simulink subsystem "dynamics"  (R2023b)
settings: Solver=VariableStepAuto  StartTime=0.0  StopTime=10.0  RelTol=1e-3
undefined symbols (not defined in the file): a, b, Cf_rad, Cr_rad, Iz, raptor_xcp_function, totalMass, Vcg
libraries: Raptor_lib x39, dynamics_lib x11, cstblocks x1, mpclib x1
settings Model: Creator=serga  LastModifiedBy=serga
settings OptimizationCC: ReuseModelBlockBuffer=off

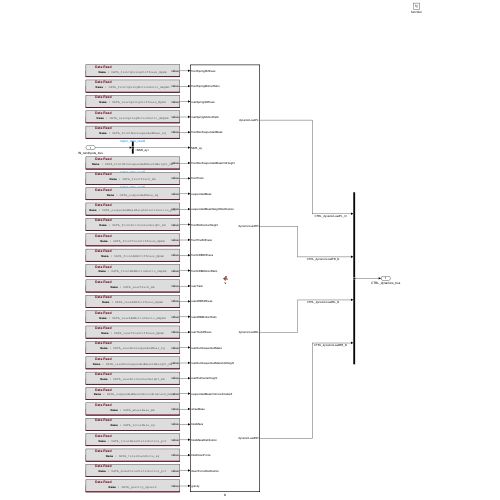
[thumbnail: Simulink's stored preview of the top-level diagram]
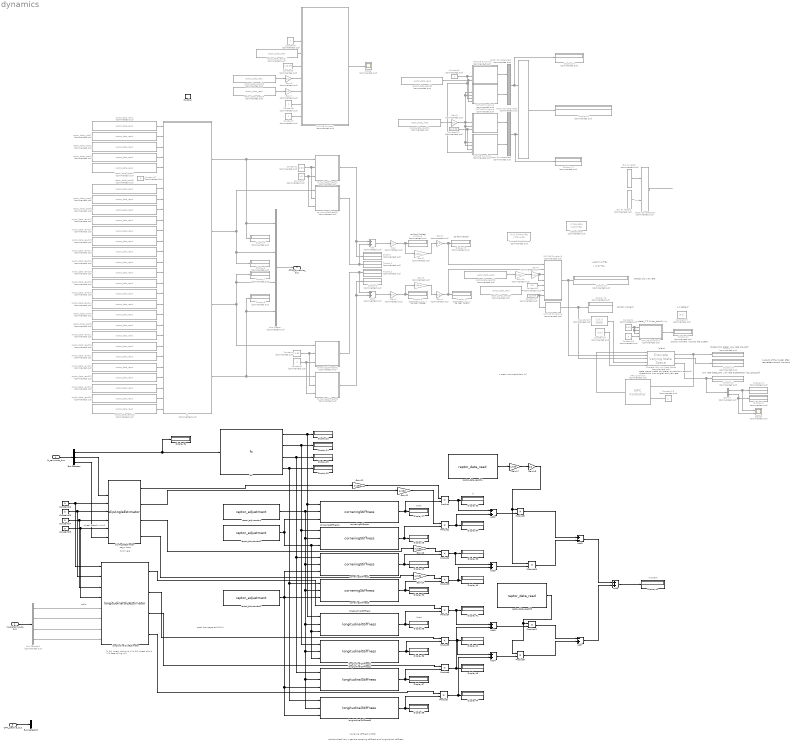
== system dynamics ==
  note: N
  note: moment
  note: peak tire usage at 0.3-0.4
  note: % full wheel lockup is -1
      | % full wheel slip is 1
      | % free rolling is 0
  note: rad/s
  note: wheel speed in km/h
  note: km/h here
  note: deg/s here
  note: double check how u get the cornering stiffness and longitudinal stiffness
  note: cornering stiffness = BCD
  note: outputs of the model after requested control moment
  note: "plant"
  note: state space model for lateral dynamics in terms of chassis slip (yaw angle) and yaw rate
  note: control moment, input to the system
  note: delta_T = Kr*psi_dot+Kv*vy
  note: chassis slip (beta), yaw rate (psi_dot)
  note: yaw rate (beta_dot), yaw rate acceleration (psi_dot_dot))
  note: u matrix as output from lu?
  note: y = Cx+Du
  note: x_dot = Ax+Bu
  note: control moment
  note: chassis slip
      | yaw rate
  note: ca rear (N/deg)
  note: ca front (N/deg)
  note: ca front (N/rad)
  note: ca rear (N/rad)
  note: u is delta_T
  note: N/rad
  note: N/rad
  IN_canInputs_bus : Inport
  IN_digitalInputs_bus : Inport  Port=2
  CTRL_tractive_bus : Inport  Port=3
  function : TriggerPort  TriggerType=function-call  VariantControl=(inherit)
  Add : Sum  Commented=on
  Add1 : Sum  Commented=on
  Add{2..5,8} (5 alike) : Sum
  Add6 : Sum  Inputs=+-
  Add7 : Sum  Inputs=-+
  Bus Creator : BusCreator  Commented=on  Inputs=4
  Bus Selector : BusSelector  OutputSignals=IN_can2Inputs_bus.CAN2_mm5_bus.CAN2_mm5_372_bus.MM5_ay,IN_can2Inputs_bus.CAN2_mm5_bus.CAN2_mm5_372_bus.MM5_yawRate,IN_can1Inputs_bus.CAN1_lws_bus.CAN1_lws_688_bus.LWS_angle
  Bus Selector1 : BusSelector  Commented=on  OutputSignals=IN_wheelSpeed_Bus.IN_wheelSpeedFL_bus.IN_wheelSpeedFL_radpsec,IN_wheelSpeed_Bus.IN_wheelSpeedFR_bus.IN_wheelSpeedFR_radpsec,IN_wheelSpeed_Bus.IN_wheelSpeedRL_bus.IN_wheelSpeedRL_radpsec,IN_wheelSpeed_Bus.IN_wheelSpeedRR_bus.IN_wheelSpeedRR_radpsec
  Bus Selector2 : BusSelector  OutputSignals=CTRL_vehicleSpeed_mph
  Bus to Vector : BusToVector  Commented=on
  Bus to Vector1 : BusToVector  Commented=on
  Constant : Constant  Commented=on  Value=0.83
  Constant{1,6..9,18} (6 alike) : Constant  Commented=on
  Constant10 : Constant  Commented=on  Value=113.95
  Constant11 : Constant  Commented=on  Value=113.95
  Constant12 : Constant  Commented=on  Value=15
  Constant13 : Constant  Commented=on  Value=[1 0; 0 10000]  VectorParams1D=off
  Constant14 : Constant  Commented=on  Value=[0;0]  VectorParams1D=off
  Constant15 : Constant  Commented=on  Value=[0.1]  VectorParams1D=off
  Constant16 : Constant  Commented=on  Value=3
  Constant17 : Constant  Commented=on  Value=0
  Constant2 : Constant  Commented=on  Value=0.83
  Constant{22..25} (4 alike) : Constant  Value=5
  Constant3 : Constant  Commented=on  Value=1.5
  Constant4 : Constant  Commented=on  Value=0.01
  Constant5 : Constant  Commented=on  Value=113.95
  Demux : Demux  Commented=on  Outputs=2
  Discrete State-Space : DiscreteStateSpace  Commented=on  SampleTime=-1
  Discrete Varying State Space : cstblocks/Linear Parameter Varying/Discrete Varying State Space  Commented=on  x0=0  Ts=-1  OutputX=on  OutputDX=on  Feedthrough=on
  Display{,1..22} (23 alike) : Display  Commented=on
  Display{23..31,33..45} (22 alike) : Display
  Gain : Gain  Commented=on  Gain=1/4
  Gain1 : Gain  Commented=on  Gain=1/4
  Gain10 : Gain  Commented=on  Gain=1/100
  Gain{11..14} (4 alike) : Gain  Gain=pi/180
  Gain17 : Gain  Gain=1/100
  Gain18 : Gain  Gain=1/2
  Gain2 : Gain  Commented=on  Gain=180/pi
  Gain3 : Gain  Commented=on  Gain=180/pi
  Gain{4..9} (6 alike) : Gain  Commented=on  Gain=1/2
  MATLAB Function : MATLAB Function  Commented=on  TreatAsAtomicUnit=on
  MATLAB Function1 : MATLAB Function  Commented=on  TreatAsAtomicUnit=on
  MATLAB Function2 : MATLAB Function  Commented=on  TreatAsAtomicUnit=on
  MATLAB Function3 : MATLAB Function  Commented=on  TreatAsAtomicUnit=on
  MATLAB Function4 : MATLAB Function  Commented=on  TreatAsAtomicUnit=on
  MATLAB Function5 : MATLAB Function  Commented=on  TreatAsAtomicUnit=on
  MATLAB Function6 : MATLAB Function  Commented=on  TreatAsAtomicUnit=on
  MATLAB Function7 : MATLAB Function  Commented=on  TreatAsAtomicUnit=on
  MPC Controller : mpclib/MPC Controller  Commented=on  SCDEnableBlockLinearizationSpecification=on  is_multiple=0  enable_value=0  return_u0=off  updateMPCinCallerWorkspace=on  md_inport=off  mv_inport=off  uref_inport=off  return_cost=off  return_mvseq=off  return_qpstatus=off  return_xseq=off  return_state=off  return_ovseq=off  state_inport=off  umin_inport=off  umax_inport=off  ymin_inport=off  ymax_inport=off  cc_inport=off  ywt_inport=off  uwt_inport=off  duwt_inport=off  rhoeps_inport=off  pm_inport=off  MaximumP=10  HorizonChoice=FixedHorizon  n_ts=0.1  n_p=10  n_mv=1  n_md=1  n_ud=0  n_mo=1  n_uo=0  BlockDataType=double  SampleTimeInherited=off  switch_inport=off
  Product{,1..11} (12 alike) : Product
  Scope : Scope  Commented=on
  Scope1 : Scope  Commented=on  NumInputPorts=2
  State-Space : StateSpace  Commented=on  A=[-(2*(Cf_rad+Cr_rad))/(Vcg*totalMass) -(2*(a*Cf_rad-b*Cr_rad))/(Vcg^2*totalMass)-1; -(2*(a*Cf_rad-2*b*Cr_rad))/Iz -(2*(a^2*Cf_rad-b^2*Cr_rad))/(Vcg*Iz)]  B=[0; 1/Iz]  C=[1 0; 0 1]  D=[0; 0]  InitialCondition=0
  Vector Concatenate : Concatenate  Commented=on  Mode=Multidimensional array  ConcatenateDimension=2
  Vector Concatenate2 : Concatenate  Commented=on
  Vector Concatenate3 : Concatenate  Commented=on
  Vector Concatenate4 : Concatenate  Commented=on  Mode=Multidimensional array  ConcatenateDimension=2
  corneringStiffness : dynamics_lib/corneringStiffness  pos='FL'
  corneringStiffness1 : dynamics_lib/corneringStiffness  pos='FR'
  corneringStiffness2 : dynamics_lib/corneringStiffness  pos='RL'
  corneringStiffness3 : dynamics_lib/corneringStiffness  pos='RR'
  corneringStiffnessFL : MATLAB Function  Commented=on  TreatAsAtomicUnit=on
  corneringStiffnessFR : MATLAB Function  Commented=on  TreatAsAtomicUnit=on
  corneringStiffnessRL : MATLAB Function  Commented=on  TreatAsAtomicUnit=on
  corneringStiffnessRR : MATLAB Function  Commented=on  TreatAsAtomicUnit=on
  fz : MATLAB Function  Commented=on  TreatAsAtomicUnit=on
  fz1 : dynamics_lib/fz  SystemSampleTime=-1  VariantActivationTime=update diagram  AllowFlexibleInterface=on  Latency=0  AutoFrameSizeCalculation=off
  longitudinalSlipEstimator : dynamics_lib/longitudinalSlipEstimator  SystemSampleTime=-1  VariantActivationTime=update diagram  AllowFlexibleInterface=on  Latency=0  AutoFrameSizeCalculation=off
  longitudinalStiffness : dynamics_lib/longitudinalStiffness  pos='FL'
  longitudinalStiffness1 : dynamics_lib/longitudinalStiffness  pos='FR'
  longitudinalStiffness2 : dynamics_lib/longitudinalStiffness  pos='RL'
  longitudinalStiffness3 : dynamics_lib/longitudinalStiffness  pos='RR'
  raptor_adjustment : Raptor_lib/Data Storage/raptor_adjustment  paramName='DATA_tirePressure_bar'  nameSource=Parameter  initValue=0.83  dataType=double  storage=Calibration  calDispType=Number  calEnum={'False', 'True'}  calGain=1.0  calOffset=0.0  calMax=inf  calMin=-inf  calFormat='-1'  calUnit=''  calHelp=''  calAccess=1  calFunction=raptor_xcp_function(gcb)  calDispHeaders=off  calColHeaders={'Col1' 'Col2' 'Col3'}  calRowHeaders={'Row1' 'Row2' 'Row3'}
      settings: SourceProductName=Raptor
  raptor_adjustment1 : Raptor_lib/Data Storage/raptor_adjustment  paramName='DATA_inclineAngleF_deg'  nameSource=Parameter  initValue=1.5  dataType=single  storage=Calibration  calDispType=Number  calEnum={'False', 'True'}  calGain=1.0  calOffset=0.0  calMax=inf  calMin=-inf  calFormat='-1'  calUnit=''  calHelp=''  calAccess=1  calFunction=raptor_xcp_function(gcb)  calDispHeaders=off  calColHeaders={'Col1' 'Col2' 'Col3'}  calRowHeaders={'Row1' 'Row2' 'Row3'}
      settings: SourceProductName=Raptor
  raptor_adjustment2 : Raptor_lib/Data Storage/raptor_adjustment  paramName='DATA_inclineAngleR_deg'  nameSource=Parameter  initValue=1  dataType=single  storage=Calibration  calDispType=Number  calEnum={'False', 'True'}  calGain=1.0  calOffset=0.0  calMax=inf  calMin=-inf  calFormat='-1'  calUnit=''  calHelp=''  calAccess=1  calFunction=raptor_xcp_function(gcb)  calDispHeaders=off  calColHeaders={'Col1' 'Col2' 'Col3'}  calRowHeaders={'Row1' 'Row2' 'Row3'}
      settings: SourceProductName=Raptor
  raptor_data_read : Raptor_lib/Data Storage/raptor_data_read  Commented=on  dataName='DATA_frontSpringStiffness_Npmm'  dataShape=Scalar  idxSource=Input  idxRow=1  idxCol=1
      settings: SourceProductName=Raptor
  raptor_data_read1 : Raptor_lib/Data Storage/raptor_data_read  Commented=on  dataName='DATA_rearSpringStiffness_Npmm'  dataShape=Scalar  idxSource=Input  idxRow=1  idxCol=1
      settings: SourceProductName=Raptor
  raptor_data_read10 : Raptor_lib/Data Storage/raptor_data_read  Commented=on  dataName='DATA_suspendedMassWeightDistribution_pct'  dataShape=Scalar  idxSource=Input  idxRow=1  idxCol=1
      settings: SourceProductName=Raptor
  raptor_data_read11 : Raptor_lib/Data Storage/raptor_data_read  Commented=on  dataName='DATA_frontRollCenterHeight_mm'  dataShape=Scalar  idxSource=Input  idxRow=1  idxCol=1
      settings: SourceProductName=Raptor
  raptor_data_read12 : Raptor_lib/Data Storage/raptor_data_read  Commented=on  dataName='DATA_rearRollCenterHeight_mm'  dataShape=Scalar  idxSource=Input  idxRow=1  idxCol=1
      settings: SourceProductName=Raptor
  raptor_data_read13 : Raptor_lib/Data Storage/raptor_data_read  Commented=on  dataName='DATA_frontTireStiffness_Npmm'  dataShape=Scalar  idxSource=Input  idxRow=1  idxCol=1
      settings: SourceProductName=Raptor
  raptor_data_read14 : Raptor_lib/Data Storage/raptor_data_read  Commented=on  dataName='DATA_rearTireStiffness_Npmm'  dataShape=Scalar  idxSource=Input  idxRow=1  idxCol=1
      settings: SourceProductName=Raptor
  raptor_data_read15 : Raptor_lib/Data Storage/raptor_data_read  Commented=on  dataName='DATA_rearARBStiffness_Npmm'  dataShape=Scalar  idxSource=Input  idxRow=1  idxCol=1
      settings: SourceProductName=Raptor
  raptor_data_read16 : Raptor_lib/Data Storage/raptor_data_read  Commented=on  dataName='DATA_frontARBMotionRatio_mmpmm'  dataShape=Scalar  idxSource=Input  idxRow=1  idxCol=1
      settings: SourceProductName=Raptor
  raptor_data_read17 : Raptor_lib/Data Storage/raptor_data_read  Commented=on  dataName='DATA_frontARBStiffness_Npmm'  dataShape=Scalar  idxSource=Input  idxRow=1  idxCol=1
      settings: SourceProductName=Raptor
  raptor_data_read18 : Raptor_lib/Data Storage/raptor_data_read  Commented=on  dataName='DATA_rearARBMotionRatio_mmpmm'  dataShape=Scalar  idxSource=Input  idxRow=1  idxCol=1
      settings: SourceProductName=Raptor
  raptor_data_read19 : Raptor_lib/Data Storage/raptor_data_read  Commented=on  dataName='DATA_rearTrack_mm'  dataShape=Scalar  idxSource=Input  idxRow=1  idxCol=1
      settings: SourceProductName=Raptor
  raptor_data_read2 : Raptor_lib/Data Storage/raptor_data_read  Commented=on  dataName='DATA_frontSpringMotionRatio_mmpmm'  dataShape=Scalar  idxSource=Input  idxRow=1  idxCol=1
      settings: SourceProductName=Raptor
  raptor_data_read20 : Raptor_lib/Data Storage/raptor_data_read  Commented=on  dataName='DATA_suspendedMassCGCoordinatesZ_mm'  dataShape=Scalar  idxSource=Input  idxRow=1  idxCol=1
      settings: SourceProductName=Raptor
  raptor_data_read{21,28..29,31..32} (5 alike) : Raptor_lib/Data Storage/raptor_data_read  Commented=on  dataName='DATA_wheelBase_mm'  dataShape=Scalar  idxSource=Input  idxRow=1  idxCol=1
      settings: SourceProductName=Raptor
  raptor_data_read{22,27,30,33} (4 alike) : Raptor_lib/Data Storage/raptor_data_read  Commented=on  dataName='DATA_totalMass_kg'  dataShape=Scalar  idxSource=Input  idxRow=1  idxCol=1
      settings: SourceProductName=Raptor
  raptor_data_read23 : Raptor_lib/Data Storage/raptor_data_read  Commented=on  dataName='DATA_totalMassDistribution_pct'  dataShape=Scalar  idxSource=Input  idxRow=1  idxCol=1
      settings: SourceProductName=Raptor
  raptor_data_read24 : Raptor_lib/Data Storage/raptor_data_read  Commented=on  dataName='DATA_totalDownForce_kg'  dataShape=Scalar  idxSource=Input  idxRow=1  idxCol=1
      settings: SourceProductName=Raptor
  raptor_data_read25 : Raptor_lib/Data Storage/raptor_data_read  Commented=on  dataName='DATA_downForceDistribution_pct'  dataShape=Scalar  idxSource=Input  idxRow=1  idxCol=1
      settings: SourceProductName=Raptor
  raptor_data_read26 : Raptor_lib/Data Storage/raptor_data_read  Commented=on  dataName='DATA_gravity_mpsec2'  dataShape=Scalar  idxSource=Input  idxRow=1  idxCol=1
      settings: SourceProductName=Raptor
  raptor_data_read3 : Raptor_lib/Data Storage/raptor_data_read  Commented=on  dataName='DATA_rearSpringMotionRatio_mmpmm'  dataShape=Scalar  idxSource=Input  idxRow=1  idxCol=1
      settings: SourceProductName=Raptor
  raptor_data_read34 : Raptor_lib/Data Storage/raptor_data_read  dataName='DATA_wheelBase_mm'  dataShape=Scalar  idxSource=Input  idxRow=1  idxCol=1
      settings: SourceProductName=Raptor
  raptor_data_read35 : Raptor_lib/Data Storage/raptor_data_read  dataName='DATA_frontTrack_mm'  dataShape=Scalar  idxSource=Input  idxRow=1  idxCol=1
      settings: SourceProductName=Raptor
  raptor_data_read4 : Raptor_lib/Data Storage/raptor_data_read  Commented=on  dataName='DATA_frontNonSuspendedMass_kg'  dataShape=Scalar  idxSource=Input  idxRow=1  idxCol=1
      settings: SourceProductName=Raptor
  raptor_data_read5 : Raptor_lib/Data Storage/raptor_data_read  Commented=on  dataName='DATA_frontNonSuspendedMassCGHeight_mm'  dataShape=Scalar  idxSource=Input  idxRow=1  idxCol=1
      settings: SourceProductName=Raptor
  raptor_data_read6 : Raptor_lib/Data Storage/raptor_data_read  Commented=on  dataName='DATA_frontTrack_mm'  dataShape=Scalar  idxSource=Input  idxRow=1  idxCol=1
      settings: SourceProductName=Raptor
  raptor_data_read7 : Raptor_lib/Data Storage/raptor_data_read  Commented=on  dataName='DATA_rearNonSuspendedMass_kg'  dataShape=Scalar  idxSource=Input  idxRow=1  idxCol=1
      settings: SourceProductName=Raptor
  raptor_data_read8 : Raptor_lib/Data Storage/raptor_data_read  Commented=on  dataName='DATA_rearNonSuspendedMassCGHeight_mm'  dataShape=Scalar  idxSource=Input  idxRow=1  idxCol=1
      settings: SourceProductName=Raptor
  raptor_data_read9 : Raptor_lib/Data Storage/raptor_data_read  Commented=on  dataName='DATA_suspendedMass_kg'  dataShape=Scalar  idxSource=Input  idxRow=1  idxCol=1
      settings: SourceProductName=Raptor
  slipAngleEstimator : dynamics_lib/slipAngleEstimator  SystemSampleTime=-1  VariantActivationTime=update diagram  AllowFlexibleInterface=on  Latency=0  AutoFrameSizeCalculation=off
  CTRL_dynamics_bus : Outport
  wires:
  fz/4(dynamicLoadRR) -> corneringStiffnessRR/1(Fz), Bus Creator/4, Display5/1  "CTRL_dynamicLoadRR_N"
  fz/3(dynamicLoadRL) -> Bus Creator/3, Display7/1, corneringStiffnessRL/1(Fz)  "CTRL_dynamicLoadRL_N"
  fz/2(dynamicLoadFR) -> corneringStiffnessFR/1(Fz), Bus Creator/2, Display6/1  "CTRL_dynamicLoadFR_N"
  fz/1(dynamicLoadFL) -> corneringStiffnessFL/1(Fz), Bus Creator/1, Display4/1  "CTRL_dynamicLoadFL_N"
  Bus Creator/1 -> CTRL_dynamics_bus/1
  raptor_data_read/1 -> fz/1(frontSpringStiffness)
  raptor_data_read1/1 -> fz/3(rearSpringStiffness)
  raptor_data_read2/1 -> fz/2(frontSpringMotionRatio)
  raptor_data_read3/1 -> fz/4(rearSpringMotionRatio)
  raptor_data_read4/1 -> fz/5(frontNonSuspendedMass)
  raptor_data_read5/1 -> fz/7(frontNonSuspendedMassCGHeight)
  raptor_data_read6/1 -> fz/8(frontTrack)
  raptor_data_read7/1 -> fz/19(rearNonSuspendedMass)
  raptor_data_read8/1 -> fz/20(rearNonSuspendedMassCGHeight)
  raptor_data_read9/1 -> fz/9(suspendedMass)
  raptor_data_read10/1 -> fz/10(suspendedMassWeightDistribution)
  raptor_data_read11/1 -> fz/11(frontRollCenterHeight)
  raptor_data_read12/1 -> fz/21(rearRollCenterHeight)
  raptor_data_read13/1 -> fz/12(frontTireStiffness)
  raptor_data_read14/1 -> fz/18(rearTireStiffness)
  raptor_data_read17/1 -> fz/13(frontARBStiffness)
  raptor_data_read18/1 -> fz/17(rearARBMotionRatio)
  raptor_data_read16/1 -> fz/14(frontARBMotionRatio)
  raptor_data_read15/1 -> fz/16(rearARBStiffness)
  raptor_data_read19/1 -> fz/15(rearTrack)
  raptor_data_read20/1 -> fz/22(suspendedMassCGCoordinatesZ)
  raptor_data_read21/1 -> fz/23(wheelBase)
  raptor_data_read22/1 -> fz/24(totalMass)
  raptor_data_read23/1 -> fz/25(totalMassDistribution)
  raptor_data_read24/1 -> fz/26(totalDownForce)
  raptor_data_read25/1 -> fz/27(downForceDistribution)
  raptor_data_read26/1 -> fz/28(gravity)
  Constant/1 -> corneringStiffnessRL/2(pressure), corneringStiffnessRR/2(pressure)
  Constant1/1 -> corneringStiffnessRL/3(inclangl), corneringStiffnessRR/3(inclangl)
  Constant2/1 -> corneringStiffnessFL/2(pressure), corneringStiffnessFR/2(pressure)
  Constant3/1 -> corneringStiffnessFL/3(inclangl), corneringStiffnessFR/3(inclangl)
  corneringStiffnessFL/1(Ca) -> Display/1, Add/1
  corneringStiffnessFR/1(Ca) -> Display1/1, Add/2
  corneringStiffnessRL/1(Ca) -> Display2/1, Add1/1
  corneringStiffnessRR/1(Ca) -> Display3/1, Add1/2
  Add1/1 -> Gain1/1
  Constant17/1 -> fz/6(MM5_ay)
  Add/1 -> Gain/1
  Gain/1 -> Display8/1, Gain2/1
  Gain1/1 -> Display9/1, Gain3/1
  Gain2/1 -> Gain5/1
  Gain3/1 -> Gain4/1
  Gain4/1 -> Display11/1, MATLAB Function5/2(Cr_rad)
  Gain5/1 -> Display10/1, MATLAB Function5/1(Cf_rad)
  Bus to Vector/1 -> Vector Concatenate/1
  Bus to Vector1/1 -> Vector Concatenate/2
  Vector Concatenate/1 -> ?  "A"
  MATLAB Function6/1(y) -> Display16/1, Discrete Varying State Space/3  "B"
  MATLAB Function5/1(y) -> Display15/1, Discrete Varying State Space/2  "A"
  MATLAB Function3/1(y) -> Vector Concatenate3/1
  Vector Concatenate4/1 -> Display12/1  "A"
  MATLAB Function1/1(y) -> Vector Concatenate2/1
  raptor_data_read30/1 -> MATLAB Function1/4(totalMass), MATLAB Function2/6(totalMass)
  raptor_data_read31/1 -> Gain8/1
  Vector Concatenate3/1 -> Vector Concatenate4/2, Display13/1
  Gain8/1 -> MATLAB Function3/4(b), MATLAB Function4/3(a), MATLAB Function4/4(b), MATLAB Function3/3(a), MATLAB Function2/4(b), MATLAB Function2/3(a)
  MATLAB Function2/1(y) -> Vector Concatenate2/2
  Constant10/1 -> MATLAB Function3/5(Iz), MATLAB Function4/5(Iz)
  Constant9/1 -> MATLAB Function4/6(Vcg), MATLAB Function2/5(Vcg), MATLAB Function1/3(Vcg)
  Vector Concatenate2/1 -> Vector Concatenate4/1, Display14/1
  MATLAB Function4/1(y) -> Vector Concatenate3/2
  raptor_data_read27/1 -> MATLAB Function/4(totalMass)
  MATLAB Function/1(syss) -> Scope/1
  Constant8/1 -> MATLAB Function/3(Vcg)
  raptor_data_read28/1 -> Gain6/1
  Constant7/1 -> MATLAB Function/9(Kv)
  Constant5/1 -> MATLAB Function/5(Iz)
  raptor_data_read29/1 -> Gain7/1
  Constant6/1 -> MATLAB Function/8(Kr)
  Gain6/1 -> MATLAB Function/6(a)
  Gain7/1 -> MATLAB Function/7(b)
  raptor_data_read32/1 -> Gain10/1
  Gain9/1 -> MATLAB Function5/3(a), MATLAB Function5/4(b)
  Constant11/1 -> MATLAB Function5/7(Iz), MATLAB Function6/1(Iz)
  Constant12/1 -> MATLAB Function5/5(Vcg)
  raptor_data_read33/1 -> MATLAB Function5/6(totalMass)
  Gain10/1 -> Gain9/1
  Constant14/1 -> Discrete Varying State Space/5  "D"
  Constant13/1 -> Discrete Varying State Space/4  "C"
  Discrete Varying State Space/1 -> Display17/1, MPC Controller/1
  Discrete Varying State Space/2 -> Display18/1
  Discrete Varying State Space/3 -> Display19/1, Demux/1
  Demux/1 -> Display20/1, Scope1/1  "yaw rate"
  Demux/2 -> Display21/1, Scope1/2  "yaw rate acceleration"
  MATLAB Function7/1(y) -> Display22/1
  Constant4/1 -> MATLAB Function7/1(Kr), MATLAB Function7/2(Kv), MATLAB Function7/3(psi_dot)
  Constant16/1 -> MATLAB Function7/4(vy)
  MPC Controller/1 -> Discrete Varying State Space/1  "control moment"
  Constant18/1 -> MPC Controller/2
  fz1/1 -> Display23/1, longitudinalStiffness/1, corneringStiffness/1
  fz1/4 -> longitudinalStiffness3/1, corneringStiffness3/1, Display26/1
  fz1/2 -> Display24/1, corneringStiffness1/1, longitudinalStiffness1/1
  fz1/3 -> Display25/1, corneringStiffness2/1, longitudinalStiffness2/1
  raptor_adjustment/1 -> corneringStiffness2/2, corneringStiffness3/2, longitudinalStiffness/2, longitudinalStiffness1/2, longitudinalStiffness2/2, longitudinalStiffness3/2, corneringStiffness1/2, corneringStiffness/2
  raptor_adjustment1/1 -> corneringStiffness/3, corneringStiffness1/3, longitudinalStiffness/3, longitudinalStiffness1/3
  raptor_adjustment2/1 -> corneringStiffness3/3, longitudinalStiffness2/3, longitudinalStiffness3/3, corneringStiffness2/3
  corneringStiffness3/1 -> Display30/1, Product3/2
  corneringStiffness2/1 -> Display29/1, Product2/2
  corneringStiffness1/1 -> Display28/1, Product1/2
  corneringStiffness/1 -> Display27/1, Product/2
  longitudinalStiffness/1 -> Display35/1, Product4/2
  longitudinalStiffness1/1 -> Display36/1, Product5/2
  longitudinalStiffness2/1 -> Display37/1, Product6/2
  longitudinalStiffness3/1 -> Display38/1, Product7/2
  IN_canInputs_bus/1 -> Bus Selector/1
  slipAngleEstimator/1 -> Gain12/1
  slipAngleEstimator/2 -> Gain11/1
  slipAngleEstimator/3 -> Gain13/1
  Constant25/1 -> slipAngleEstimator/6, longitudinalSlipEstimator/4
  Constant24/1 -> slipAngleEstimator/5, longitudinalSlipEstimator/3
  Constant23/1 -> slipAngleEstimator/4, longitudinalSlipEstimator/2
  Constant22/1 -> slipAngleEstimator/3, longitudinalSlipEstimator/1
  Product/1 -> Display33/1, Add2/1
  Product1/1 -> Display34/1, Add2/2
  Product2/1 -> Display39/1, Add3/1
  Product3/1 -> Display40/1, Add3/2
  Product4/1 -> Display41/1, Add5/1
  Product5/1 -> Display42/1, Add4/1
  Product6/1 -> Display43/1, Add5/2
  Product7/1 -> Display44/1, Add4/2
  Gain11/1 -> Product1/1
  Gain12/1 -> Product/1
  Gain13/1 -> Product2/1
  slipAngleEstimator/4 -> Gain14/1
  Gain14/1 -> Product3/1
  Add2/1 -> Product8/2
  Add3/1 -> Product10/2
  Add4/1 -> Product9/2
  Add5/1 -> Product11/2
  raptor_data_read34/1 -> Gain17/1
  Gain17/1 -> Gain18/1
  Gain18/1 -> Product10/1, Product8/1
  raptor_data_read35/1 -> Product11/1, Product9/1
  Product8/1 -> Add6/1
  Product10/1 -> Add6/2
  Product11/1 -> Add7/1
  Product9/1 -> Add7/2
  Add6/1 -> Add8/1
  Add7/1 -> Add8/2
  Add8/1 -> Display45/1
  longitudinalSlipEstimator/1 -> Product4/1
  longitudinalSlipEstimator/2 -> Product5/1
  longitudinalSlipEstimator/3 -> Product6/1
  longitudinalSlipEstimator/4 -> Product7/1
  IN_digitalInputs_bus/1 -> Bus Selector1/1
  Bus Selector1/1 -> longitudinalSlipEstimator/5  "<IN_wheelSpeedFL_radpsec>"
  Bus Selector1/2 -> longitudinalSlipEstimator/6  "<IN_wheelSpeedFR_radpsec>"
  Bus Selector1/3 -> longitudinalSlipEstimator/7  "<IN_wheelSpeedRL_radpsec>"
  Bus Selector1/4 -> longitudinalSlipEstimator/8  "<IN_wheelSpeedRR_radpsec>"
  Bus Selector/1 -> fz1/1, Display31/1  "<MM5_ay>"
  Bus Selector/2 -> slipAngleEstimator/2  "<MM5_yawRate>"
  Bus Selector/3 -> slipAngleEstimator/7  "<LWS_angle>"
  CTRL_tractive_bus/1 -> Bus Selector2/1

== matlab function dynamics/corneringStiffnessRR ==
  data: Fz input; Ca output; pressure input; inclangl input
function Ca = fcn(Fz,pressure,inclangl)
FNOMIN = 1100;
LFZO = 1;
NOMPRES = 96500;
LCY = 1;
PCY1 = 1.5666;
PDY1 = 2.2511;
PDY2 = -0.0605;
PPY3 = 0.0842; 
PPY4 = 0.0577;
PDY3 = 0.0764;
LMUY = 1; 
PKY1 = -23.4258; 
PPY1 = -1.2848;
PKY3 = 0.1036;
PKY4 = 2.000;
PKY2 = 1.1000; 
PKY5 = 2.9328; 
PPY2 = -1.0252;
LKY = 1;
% LKYC = 1;
% PVY3 = 0.8518;
% PVY4 = 0.6702;
% PKY6 = -2.8877;
% PKY7 = -0.8116;
% PPY5 =  -2.0029;
% LVY = 1;
% PVY1 = 0.0394;
% PVY2 = -0.0391;
% LHY = 1;
% PHY1 = 0.0004; 
% PHY2 = 0.0005;
% PEY1 = -0.4203;
% PEY2 = -1.0400;
% PEY5 = 0.0032;
% PEY3 = -0.5785;
% PEY4 = 0.0857;
% LEY = 1; 
% 
% ZETA0 = 1;
ZETA2 = 1;
ZETA3 = 1;
% ZETA4 = 1;

gammaAst = sin(inclangl); 
gammaAst2 = gammaAst.^2;    

Fz0_ = FNOMIN.*LFZO; 

dfz = (Fz-Fz0_)./Fz0_; 
 
pi0 = NOMPRES; 
dpi = (pressure-pi0)./pi0; 
dpi2 = dpi.^2; 

Cy = LCY.*PCY1; 

muy = (PDY1+PDY2.*dfz).*(1+PPY3.*dpi+PPY4.*dpi2)... 
    .*(1-PDY3.*gammaAst2).*LMUY;

Dy = muy.*Fz.*ZETA2; 

Kya = PKY1.*Fz0_... 
    .*(1+PPY1.*dpi)...
    .*(1-PKY3.*abs(gammaAst))...
    .*sin(PKY4.*atan(Fz./Fz0_./((PKY2+PKY5.*gammaAst2)...
    .*(1+PPY2.*dpi)))).*LKY.*ZETA3;

Ca = -Kya;

== matlab function dynamics/MATLAB Function ==
  data: Cf_rad input; syss output; Cr_rad input; Vcg input; totalMass input; Iz input; a input; b input; Kr input; Kv input
function syss = fcn(Cf_rad, Cr_rad, Vcg, totalMass, Iz, a, b, Kr, Kv)

A = [-(2*(Cf_rad+Cr_rad))/(Vcg*totalMass) -(2*(a*Cf_rad-b*Cr_rad))/(Vcg^2*totalMass)-1; ...
     -(2*(a*Cf_rad-2*b*Cr_rad))/Iz        -(2*(a^2*Cf_rad-b^2*Cr_rad))/(Vcg*Iz)];

B = [0; ...
     1/Iz];

% Kr = 1;
% Kv = 1;

delta_T = Kr*psi_dot+Kv*vy; 

C = eye(2);

D = zeros(2,1);

% discretized state space
sys = ss(A,B,C,D,-1);

Q = [1 0; ...
     0 1000];

% Q = C'*C

% R = 0.1
R = 0.001;

[K,S,P] = lqr(sys,Q,R);

syss = ss(A-B*K,B,C,D);

== matlab function dynamics/MATLAB Function1 ==
  data: Cf_rad input; y output; Cr_rad input; Vcg input; totalMass input
function y = fcn(Cf_rad,Cr_rad,Vcg,totalMass)

y = -(2*(Cf_rad+Cr_rad))/(Vcg*totalMass);

== matlab function dynamics/MATLAB Function2 ==
  data: Cf_rad input; y output; Cr_rad input; a input; b input; Vcg input; totalMass input
function y = fcn(Cf_rad,Cr_rad,a,b,Vcg,totalMass)

y = -(2*(a*Cf_rad-b*Cr_rad))/(Vcg^2*totalMass)-1;

== matlab function dynamics/MATLAB Function3 ==
  data: Cf_rad input; y output; Cr_rad input; a input; b input; Iz input
function y = fcn(Cf_rad,Cr_rad,a,b,Iz)

y = -(2*(a*Cf_rad-2*b*Cr_rad))/Iz;

== matlab function dynamics/MATLAB Function4 ==
  data: Cf_rad input; y output; Cr_rad input; a input; b input; Iz input; Vcg input
function y = fcn(Cf_rad,Cr_rad,a,b,Iz,Vcg)

y = -(2*(a^2*Cf_rad-b^2*Cr_rad))/(Vcg*Iz);

== matlab function dynamics/MATLAB Function5 ==
  data: Cf_rad input; y output; Cr_rad input; a input; b input; Vcg input; totalMass input; Iz input
function y = fcn(Cf_rad,Cr_rad,a,b,Vcg,totalMass,Iz)

y = [-(2*(Cf_rad+Cr_rad))/(Vcg*totalMass) -(2*(a*Cf_rad-b*Cr_rad))/(Vcg^2*totalMass)-1; ...
     -(2*(a*Cf_rad-2*b*Cr_rad))/Iz        -(2*(a^2*Cf_rad-b^2*Cr_rad))/(Vcg*Iz)];

== matlab function dynamics/MATLAB Function6 ==
  data: Iz input; y output
function y = fcn(Iz)

y = [0; ...
     1/Iz];

== matlab function dynamics/MATLAB Function7 ==
  data: Kr input; y output; Kv input; psi_dot input; vy input
function y = fcn(Kr,Kv,psi_dot,vy)

y = Kr*psi_dot+Kv*vy;

== matlab function dynamics/fz ==
  data: frontSpringStiffness input; dynamicLoadFL output; frontSpringMotionRatio input; rearSpringStiffness input; rearSpringMotionRatio input; frontNonSuspendedMass input; MM5_ay input; frontNonSuspendedMassCGHeight input; frontTrack input; suspendedMass input; suspendedMassWeightDistribution input; frontRollCenterHeight input; frontTireStiffness input; frontARBStiffness input; frontARBMotionRatio input; rearTrack input; rearARBStiffness input; rearARBMotionRatio input; rearTireStiffness input; rearNonSuspendedMass input; rearNonSuspendedMassCGHeight input; rearRollCenterHeight input; suspendedMassCGCoordinatesZ input; wheelBase input; totalMass input; totalMassDistribution input; totalDownForce input; downForceDistribution input; gravity input; dynamicLoadFR output; dynamicLoadRL output; dynamicLoadRR output
function [dynamicLoadFL, dynamicLoadFR, dynamicLoadRL, dynamicLoadRR] = ...
    fz(frontSpringStiffness, frontSpringMotionRatio, ...
    rearSpringStiffness, rearSpringMotionRatio, frontNonSuspendedMass, ...
    MM5_ay, frontNonSuspendedMassCGHeight, frontTrack, suspendedMass, ...
    suspendedMassWeightDistribution, frontRollCenterHeight, ...
    frontTireStiffness, frontARBStiffness, frontARBMotionRatio, ...
    rearTrack, rearARBStiffness, rearARBMotionRatio, ...
    rearTireStiffness, rearNonSuspendedMass, ...
    rearNonSuspendedMassCGHeight, rearRollCenterHeight, ...
    suspendedMassCGCoordinatesZ, wheelBase, totalMass, ...
    totalMassDistribution, totalDownForce, downForceDistribution, gravity)



frontWheelRate = frontSpringStiffness/frontSpringMotionRatio^2;
rearWheelRate = rearSpringStiffness/rearSpringMotionRatio^2;
frontNSMWT = frontNonSuspendedMass*2*MM5_ay*...
    frontNonSuspendedMassCGHeight/frontTrack;
frontGeoWT = suspendedMass*(suspendedMassWeightDistribution/100)*MM5_ay*...
    frontRollCenterHeight/frontTrack;
antiRollFrontTires = ((frontTrack/1000)^2*tan(1)*frontTireStiffness* ...
    1000)/2;
antiRollFrontARB = (frontARBStiffness*1000*(frontTrack/1000)^2*tan(1))/...
    frontARBMotionRatio^2;
antiRollFrontSprings = ((frontTrack/1000)^2*tan(1)* ...
    (frontWheelRate*1000))/2;
antiRollRearSprings = ((rearTrack/1000)^2*tan(1)* ...
    (rearWheelRate*1000))/2;
antiRollRearARB = (rearARBStiffness*1000*(rearTrack/1000)^2*tan(1))/...
    rearARBMotionRatio^2;
antiRollRearTires = ((rearTrack/1000)^2*tan(1)*rearTireStiffness* ...
    1000)/2;
rearNSMWT = rearNonSuspendedMass*2*MM5_ay*...
    rearNonSuspendedMassCGHeight/rearTrack;
rearGeoWT = (suspendedMass*((100-suspendedMassWeightDistribution)/100))*...
    MM5_ay*rearRollCenterHeight/rearTrack;
deltaZ = suspendedMassCGCoordinatesZ-...
    (((rearRollCenterHeight-frontRollCenterHeight)/wheelBase* ...
        ((100-suspendedMassWeightDistribution)/100*wheelBase))+ ...
            frontRollCenterHeight);
antiRollFrontAxleAndTire = ((antiRollFrontSprings+antiRollFrontARB)* ...
    antiRollFrontTires)/((antiRollFrontSprings+antiRollFrontARB)+ ...
        antiRollFrontTires);
antiRollRearAxleAndTire = ((antiRollRearSprings+antiRollRearARB)* ...
    antiRollRearTires)/((antiRollRearSprings+antiRollRearARB)+ ...
        antiRollRearTires);
antiRollTotal = antiRollFrontAxleAndTire+antiRollRearAxleAndTire;
frontElWT = (suspendedMass*MM5_ay*deltaZ* ...
    (antiRollFrontAxleAndTire/antiRollTotal))/frontTrack;
rearElWT = (suspendedMass*MM5_ay*deltaZ* ...
    (antiRollRearAxleAndTire/antiRollTotal))/rearTrack;
frontTotalWT = frontNSMWT+frontElWT+frontGeoWT;
rearTotalWT = rearNSMWT+rearElWT+rearGeoWT;
dynamicLoadFL = (totalMass*totalMassDistribution/100*0.5+totalDownForce*...
    downForceDistribution/100/2-frontTotalWT)*gravity;
dynamicLoadFR = (totalMass*totalMassDistribution/100*0.5+totalDownForce*...
    downForceDistribution/100/2+frontTotalWT)*gravity;
dynamicLoadRL = (totalMass*(100-totalMassDistribution)/100*0.5+ ...
    totalDownForce*(100-downForceDistribution)/100/2-rearTotalWT)*gravity;
dynamicLoadRR = (totalMass*(100-totalMassDistribution)/100*0.5+ ...
    totalDownForce*(100-downForceDistribution)/100/2+rearTotalWT)*gravity;

== matlab function dynamics/corneringStiffnessFL ==
  data: Fz input; Ca output; pressure input; inclangl input
function Ca = fcn(Fz,pressure,inclangl)
FNOMIN = 1100;
LFZO = 1;
NOMPRES = 96500;
LCY = 1;
PCY1 = 1.5666;
PDY1 = 2.2511;
PDY2 = -0.0605;
PPY3 = 0.0842; 
PPY4 = 0.0577;
PDY3 = 0.0764;
LMUY = 1; 
PKY1 = -23.4258; 
PPY1 = -1.2848;
PKY3 = 0.1036;
PKY4 = 2.000;
PKY2 = 1.1000; 
PKY5 = 2.9328; 
PPY2 = -1.0252;
LKY = 1;
% LKYC = 1;
% PVY3 = 0.8518;
% PVY4 = 0.6702;
% PKY6 = -2.8877;
% PKY7 = -0.8116;
% PPY5 =  -2.0029;
% LVY = 1;
% PVY1 = 0.0394;
% PVY2 = -0.0391;
% LHY = 1;
% PHY1 = 0.0004; 
% PHY2 = 0.0005;
% PEY1 = -0.4203;
% PEY2 = -1.0400;
% PEY5 = 0.0032;
% PEY3 = -0.5785;
% PEY4 = 0.0857;
% LEY = 1; 
% 
% ZETA0 = 1;
ZETA2 = 1;
ZETA3 = 1;
% ZETA4 = 1;

gammaAst = sin(inclangl); 
gammaAst2 = gammaAst.^2;    

Fz0_ = FNOMIN.*LFZO; 

dfz = (Fz-Fz0_)./Fz0_; 
 
pi0 = NOMPRES; 
dpi = (pressure-pi0)./pi0; 
dpi2 = dpi.^2; 

Cy = LCY.*PCY1; 

muy = (PDY1+PDY2.*dfz).*(1+PPY3.*dpi+PPY4.*dpi2)... 
    .*(1-PDY3.*gammaAst2).*LMUY;

Dy = muy.*Fz.*ZETA2; 

Kya = PKY1.*Fz0_... 
    .*(1+PPY1.*dpi)...
    .*(1-PKY3.*abs(gammaAst))...
    .*sin(PKY4.*atan(Fz./Fz0_./((PKY2+PKY5.*gammaAst2)...
    .*(1+PPY2.*dpi)))).*LKY.*ZETA3;

Ca = -Kya;

== matlab function dynamics/corneringStiffnessFR ==
  data: Fz input; Ca output; pressure input; inclangl input
function Ca = fcn(Fz,pressure,inclangl)
FNOMIN = 1100;
LFZO = 1;
NOMPRES = 96500;
LCY = 1;
PCY1 = 1.5666;
PDY1 = 2.2511;
PDY2 = -0.0605;
PPY3 = 0.0842; 
PPY4 = 0.0577;
PDY3 = 0.0764;
LMUY = 1; 
PKY1 = -23.4258; 
PPY1 = -1.2848;
PKY3 = 0.1036;
PKY4 = 2.000;
PKY2 = 1.1000; 
PKY5 = 2.9328; 
PPY2 = -1.0252;
LKY = 1;
% LKYC = 1;
% PVY3 = 0.8518;
% PVY4 = 0.6702;
% PKY6 = -2.8877;
% PKY7 = -0.8116;
% PPY5 =  -2.0029;
% LVY = 1;
% PVY1 = 0.0394;
% PVY2 = -0.0391;
% LHY = 1;
% PHY1 = 0.0004; 
% PHY2 = 0.0005;
% PEY1 = -0.4203;
% PEY2 = -1.0400;
% PEY5 = 0.0032;
% PEY3 = -0.5785;
% PEY4 = 0.0857;
% LEY = 1; 
% 
% ZETA0 = 1;
ZETA2 = 1;
ZETA3 = 1;
% ZETA4 = 1;

gammaAst = sin(inclangl); 
gammaAst2 = gammaAst.^2;    

Fz0_ = FNOMIN.*LFZO; 

dfz = (Fz-Fz0_)./Fz0_; 
 
pi0 = NOMPRES; 
dpi = (pressure-pi0)./pi0; 
dpi2 = dpi.^2; 

Cy = LCY.*PCY1; 

muy = (PDY1+PDY2.*dfz).*(1+PPY3.*dpi+PPY4.*dpi2)... 
    .*(1-PDY3.*gammaAst2).*LMUY;

Dy = muy.*Fz.*ZETA2; 

Kya = PKY1.*Fz0_... 
    .*(1+PPY1.*dpi)...
    .*(1-PKY3.*abs(gammaAst))...
    .*sin(PKY4.*atan(Fz./Fz0_./((PKY2+PKY5.*gammaAst2)...
    .*(1+PPY2.*dpi)))).*LKY.*ZETA3;

Ca = -Kya;

== matlab function dynamics/corneringStiffnessRL ==
  data: Fz input; Ca output; pressure input; inclangl input
function Ca = fcn(Fz,pressure,inclangl)
FNOMIN = 1100;
LFZO = 1;
NOMPRES = 96500;
LCY = 1;
PCY1 = 1.5666;
PDY1 = 2.2511;
PDY2 = -0.0605;
PPY3 = 0.0842; 
PPY4 = 0.0577;
PDY3 = 0.0764;
LMUY = 1; 
PKY1 = -23.4258; 
PPY1 = -1.2848;
PKY3 = 0.1036;
PKY4 = 2.000;
PKY2 = 1.1000; 
PKY5 = 2.9328; 
PPY2 = -1.0252;
LKY = 1;
% LKYC = 1;
% PVY3 = 0.8518;
% PVY4 = 0.6702;
% PKY6 = -2.8877;
% PKY7 = -0.8116;
% PPY5 =  -2.0029;
% LVY = 1;
% PVY1 = 0.0394;
% PVY2 = -0.0391;
% LHY = 1;
% PHY1 = 0.0004; 
% PHY2 = 0.0005;
% PEY1 = -0.4203;
% PEY2 = -1.0400;
% PEY5 = 0.0032;
% PEY3 = -0.5785;
% PEY4 = 0.0857;
% LEY = 1; 
% 
% ZETA0 = 1;
ZETA2 = 1;
ZETA3 = 1;
% ZETA4 = 1;

gammaAst = sin(inclangl); 
gammaAst2 = gammaAst.^2;    

Fz0_ = FNOMIN.*LFZO; 

dfz = (Fz-Fz0_)./Fz0_; 
 
pi0 = NOMPRES; 
dpi = (pressure-pi0)./pi0; 
dpi2 = dpi.^2; 

Cy = LCY.*PCY1; 

muy = (PDY1+PDY2.*dfz).*(1+PPY3.*dpi+PPY4.*dpi2)... 
    .*(1-PDY3.*gammaAst2).*LMUY;

Dy = muy.*Fz.*ZETA2; 

Kya = PKY1.*Fz0_... 
    .*(1+PPY1.*dpi)...
    .*(1-PKY3.*abs(gammaAst))...
    .*sin(PKY4.*atan(Fz./Fz0_./((PKY2+PKY5.*gammaAst2)...
    .*(1+PPY2.*dpi)))).*LKY.*ZETA3;

Ca = -Kya;
